simulink model "CF017A_GmVehPwrMod"  (R2013b)
settings: Solver=FixedStepDiscrete  SolverMode=SingleTasking  StartTime=0.0  StopTime=2  FixedStep=0.002  RelTol=1e-3
values from neighbouring files (symbols this model uses):
  ASSIKEEPMINIDX_CNT_U16 = DataDict.Constant    [CF017A_GmVehPwrMod_DataDict.m]
  BUSOFFHISPDIDX_CNT_U16 = DataDict.Constant    [CF017A_GmVehPwrMod_DataDict.m]
  CNTTOSEC_ULS_U32 = DataDict.Constant    [CF017A_GmVehPwrMod_DataDict.m]
  ENGRUNACTVIDX_CNT_U16 = DataDict.Constant    [CF017A_GmVehPwrMod_DataDict.m]
  GmVehPwrModHwTqMinKeepAssi = DataDict.Calibration    [CF017A_GmVehPwrMod_DataDict.m]
  GmVehPwrModHwTqMinKeepTmr = DataDict.Calibration    [CF017A_GmVehPwrMod_DataDict.m]
  GmVehPwrModOperRampRate = DataDict.Calibration    [CF017A_GmVehPwrMod_DataDict.m]
  GMVEHPWRMODSYSSTREQENA_CNT_LOGL = DataDict.Constant    [CF017A_GmVehPwrMod_DataDict.m]
  GMVEHPWRMODVAREFF_CNT_LOGL = DataDict.Constant    [CF017A_GmVehPwrMod_DataDict.m]
  GmVehPwrModVehSpdAssiOnMin = DataDict.Calibration    [CF017A_GmVehPwrMod_DataDict.m]
  GmVehPwrModVehSpdMinKeepAssi = DataDict.Calibration    [CF017A_GmVehPwrMod_DataDict.m]
  GPIOMCUENAIDX_CNT_U16 = DataDict.Constant    [CF017A_GmVehPwrMod_DataDict.m]
  KEEPASSIIDX_CNT_U16 = DataDict.Constant    [CF017A_GmVehPwrMod_DataDict.m]
  MSG0C9MISSIDX_CNT_U16 = DataDict.Constant    [CF017A_GmVehPwrMod_DataDict.m]
  MSG1F1MISSIDX_CNT_U16 = DataDict.Constant    [CF017A_GmVehPwrMod_DataDict.m]
  SYSPWRMODRUNIDX_CNT_U16 = DataDict.Constant    [CF017A_GmVehPwrMod_DataDict.m]
  VEHSPDSNSRVLDIDX_CNT_U16 = DataDict.Constant    [CF017A_GmVehPwrMod_DataDict.m]
libraries: simulink x2, NxtrLim x2, NxtrAbslt x1
(part 4 of 4)

== system CF017A_GmVehPwrMod/GmVehPwrMod/GmVehPwrModPer1/SysStReqEna_LookupTbl_KeepOn_OnToOff/KeepAssi_Bit0/Bit0_1 ==
  Action Port : ActionPort  ActionType=then
  Constant : Constant  Value=KEEPASSIIDX_CNT_U16  OutDataTypeStr=uint16
  CopyRight2 : Subsystem  Description=|  mask(Copyright Information){none=on}
      | Copyright info block.                                               
      |                                                                     
      | Place copyright information at the top of every subsystem in design.
      mask prompts: none "No parameters"
      mask help: Place copyright information at the top of every subsystem in design.
      mask Display:
      | NxtrConf = 'Nexteer Confidential';
      | 
      | sys = bdroot; %handle for the current model ("system")
      | first = get_param(sys,'Created');
      | if(isempty(first))
      |     first = datestr(now,'yyyy');
      | else
      |     first = first(end-3:end);  %year is last four digits
      | end
      | 
      | last = get_param(sys,'LastModifiedDate');
      | if isempty(last)
      |     last = datestr(now,'yyyy');
      | else
      |     last = last(end-3:end);
      | end
      | 
      | if strcmp(first,last)
      |     fprintf('%s -- Copyright %s Nexteer',NxtrConf,first)
      | else
      |     fprintf('%s -- %s%s- %s Nexteer',NxtrConf,char(169),first,last)
      | end
  Bit0Sts : Outport
  wires:
  Constant/1 -> Bit0Sts/1

== system CF017A_GmVehPwrMod/GmVehPwrMod/GmVehPwrModPer1/SysStReqEna_LookupTbl_KeepOn_OnToOff/KeepAssi_Bit0/CopyRight2 ==

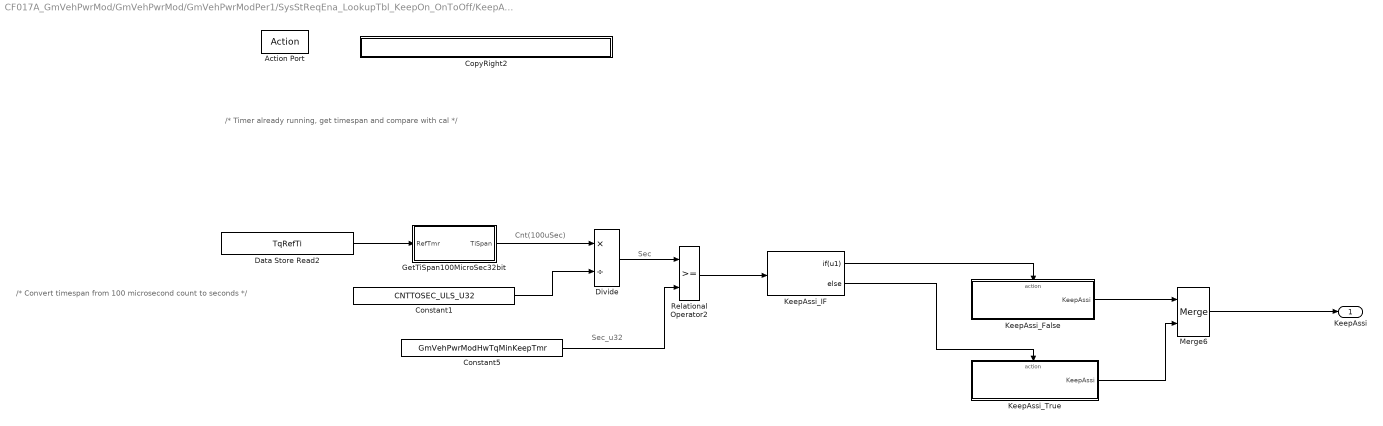
== system CF017A_GmVehPwrMod/GmVehPwrMod/GmVehPwrModPer1/SysStReqEna_LookupTbl_KeepOn_OnToOff/KeepAssi_HwTqTmr/Get_SpanTi ==
  note: Sec
  note: Cnt(100uSec)
  note: Sec_u32
  note: /* Timer already running, get timespan and compare with cal */
  note: /* Convert timespan from 100 microsecond count to seconds */
  Action Port : ActionPort  ActionType=elseif
  Constant1 : Constant  RequirementInfo={} %GIDa_aa9cc0f8_f214_4efc_ab36_0ac5a280fabf  Value=CNTTOSEC_ULS_U32  OutDataTypeStr=uint32
      settings: AttributesFormatString=%<OutDataTypeStr>
  Constant5 : Constant  RequirementInfo={} %GIDa_69eca624_6dc5_4cb0_ae9b_e1684d9a1446  Value=GmVehPwrModHwTqMinKeepTmr  OutDataTypeStr=uint32
      settings: AttributesFormatString=%<OutDataTypeStr>
  CopyRight2 : Subsystem  Description=|  mask(Copyright Information){none=on}
      | Copyright info block.                                               
      |                                                                     
      | Place copyright information at the top of every subsystem in design.
      mask prompts: none "No parameters"
      mask help: Place copyright information at the top of every subsystem in design.
      mask Display:
      | NxtrConf = 'Nexteer Confidential';
      | 
      | sys = bdroot; %handle for the current model ("system")
      | first = get_param(sys,'Created');
      | if(isempty(first))
      |     first = datestr(now,'yyyy');
      | else
      |     first = first(end-3:end);  %year is last four digits
      | end
      | 
      | last = get_param(sys,'LastModifiedDate');
      | if isempty(last)
      |     last = datestr(now,'yyyy');
      | else
      |     last = last(end-3:end);
      | end
      | 
      | if strcmp(first,last)
      |     fprintf('%s -- Copyright %s Nexteer',NxtrConf,first)
      | else
      |     fprintf('%s -- %s%s- %s Nexteer',NxtrConf,char(169),first,last)
      | end
  Data Store Read2 : DataStoreRead  DataStoreName=TqRefTi
  Divide : Product  Inputs=*/
  GetTiSpan100MicroSec32bit : Subsystem
  KeepAssi_False : Subsystem  RequirementInfo={} %GIDa_fe66f275_3ea7_40ce_bfac_a984a6fb9f78  TreatAsAtomicUnit=on
  KeepAssi_IF : If  RequirementInfo={} %GIDa_702726b2_9a9c_48b8_b9c7_15ecbfb5f8b5  IfExpression=u1
      settings: AttributesFormatString=%<Priority>
  KeepAssi_True : Subsystem  RequirementInfo={} %GIDa_583d1404_53f3_46f6_93fc_f6a44d321467  TreatAsAtomicUnit=on
  Merge6 : Merge  RequirementInfo={} %GIDa_2056328d_8088_4a66_9c76_ebdd3fb75faf
  Relational Operator2 : RelationalOperator  OutDataTypeStr=boolean
  "KeepAssi " : Outport  RequirementInfo={} %GIDa_500dc0bc_1ae5_4157_a4dd_5d2ae0a6ca5d
  wires:
  Data Store Read2/1 -> GetTiSpan100MicroSec32bit/1(RefTmr)
  Constant5/1 -> Relational Operator2/2
  GetTiSpan100MicroSec32bit/1(TiSpan) -> Divide/1
  Relational Operator2/1 -> KeepAssi_IF/1
  KeepAssi_IF/1 -> KeepAssi_False/Action
  KeepAssi_IF/2 -> KeepAssi_True/Action
  KeepAssi_False/1("KeepAssi ") -> Merge6/1
  KeepAssi_True/1("KeepAssi ") -> Merge6/2
  Constant1/1 -> Divide/2
  Divide/1 -> Relational Operator2/1
  Merge6/1 -> "KeepAssi "/1

== system CF017A_GmVehPwrMod/GmVehPwrMod/GmVehPwrModPer1/SysStReqEna_LookupTbl_KeepOn_OnToOff/KeepAssi_HwTqTmr/Stop_Tmr ==
  note: /* * Turn timer off since absolute value of handwheel torque is no longer less than HwTqMinKeepAssi cal. */
  Action Port : ActionPort  ActionType=else
  Constant1 : Constant  RequirementInfo={} %GIDa_143b7973_8004_4f87_9c2d_0949d74a0751  Value=false  OutDataTypeStr=boolean
      settings: AttributesFormatString=%<OutDataTypeStr>
  Constant4 : Constant  RequirementInfo={} %GIDa_c94d2a82_6aa0_4b23_8705_fa1f20d4de3f  Value=true  OutDataTypeStr=boolean
      settings: AttributesFormatString=%<OutDataTypeStr>
  CopyRight2 : Subsystem  Description=|  mask(Copyright Information){none=on}
      | Copyright info block.                                               
      |                                                                     
      | Place copyright information at the top of every subsystem in design.
      mask prompts: none "No parameters"
      mask help: Place copyright information at the top of every subsystem in design.
      mask Display:
      | NxtrConf = 'Nexteer Confidential';
      | 
      | sys = bdroot; %handle for the current model ("system")
      | first = get_param(sys,'Created');
      | if(isempty(first))
      |     first = datestr(now,'yyyy');
      | else
      |     first = first(end-3:end);  %year is last four digits
      | end
      | 
      | last = get_param(sys,'LastModifiedDate');
      | if isempty(last)
      |     last = datestr(now,'yyyy');
      | else
      |     last = last(end-3:end);
      | end
      | 
      | if strcmp(first,last)
      |     fprintf('%s -- Copyright %s Nexteer',NxtrConf,first)
      | else
      |     fprintf('%s -- %s%s- %s Nexteer',NxtrConf,char(169),first,last)
      | end
  Data Store Write2 : DataStoreWrite  DataStoreName=TqRefTiActv
      settings: AttributesFormatString=%<Priority>
  "KeepAssi " : Outport  RequirementInfo={} %GIDa_99310702_14e0_41e3_9d7b_f2280936931a
  wires:
  Constant1/1 -> Data Store Write2/1
  Constant4/1 -> "KeepAssi "/1

== system CF017A_GmVehPwrMod/GmVehPwrMod/GmVehPwrModPer1/SysStReqEna_LookupTbl_KeepOn_OnToOff/KeepAssi_HwTqTmr/Tmr_Strt ==
  note: /* HwTq dipped below minimum needed to keep assist and timer not yet active so start the timer now. */
  Action Port : ActionPort  ActionType=then
  Constant1 : Constant  RequirementInfo={} %GIDa_b7fdb1af_31c1_494c_99c2_7093c5cc2f63  Value=true  OutDataTypeStr=boolean
      settings: AttributesFormatString=%<OutDataTypeStr>
  Constant4 : Constant  RequirementInfo={} %GIDa_ab99e30b_c1a7_4330_836d_a1e94e7d5cba  Value=true  OutDataTypeStr=boolean
      settings: AttributesFormatString=%<OutDataTypeStr>
  CopyRight2 : Subsystem  Description=|  mask(Copyright Information){none=on}
      | Copyright info block.                                               
      |                                                                     
      | Place copyright information at the top of every subsystem in design.
      mask prompts: none "No parameters"
      mask help: Place copyright information at the top of every subsystem in design.
      mask Display:
      | NxtrConf = 'Nexteer Confidential';
      | 
      | sys = bdroot; %handle for the current model ("system")
      | first = get_param(sys,'Created');
      | if(isempty(first))
      |     first = datestr(now,'yyyy');
      | else
      |     first = first(end-3:end);  %year is last four digits
      | end
      | 
      | last = get_param(sys,'LastModifiedDate');
      | if isempty(last)
      |     last = datestr(now,'yyyy');
      | else
      |     last = last(end-3:end);
      | end
      | 
      | if strcmp(first,last)
      |     fprintf('%s -- Copyright %s Nexteer',NxtrConf,first)
      | else
      |     fprintf('%s -- %s%s- %s Nexteer',NxtrConf,char(169),first,last)
      | end
  Data Store Write1 : DataStoreWrite  DataStoreName=TqRefTi
      settings: AttributesFormatString=%<Priority>
  Data Store Write2 : DataStoreWrite  DataStoreName=TqRefTiActv
      settings: AttributesFormatString=%<Priority>
  GetRefTmr100MicroSec32bit1 : Subsystem
  "KeepAssi " : Outport  RequirementInfo={} %GIDa_aae598dd_8360_4797_8d07_5dbb83386652
  wires:
  Constant4/1 -> Data Store Write2/1
  GetRefTmr100MicroSec32bit1/1(RefTmr) -> Data Store Write1/1
  Constant1/1 -> "KeepAssi "/1

== system CF017A_GmVehPwrMod/GmVehPwrMod/GmVehPwrModPer1/SysStReqEna_LookupTbl_KeepOn_OnToOff/Msg0C9Missa_Bit4/Bit4_0 ==
  Action Port : ActionPort  ActionType=else
  Constant1 : Constant  Value=0  OutDataTypeStr=uint16
      settings: AttributesFormatString=%<OutDataTypeStr>
  CopyRight2 : Subsystem  Description=|  mask(Copyright Information){none=on}
      | Copyright info block.                                               
      |                                                                     
      | Place copyright information at the top of every subsystem in design.
      mask prompts: none "No parameters"
      mask help: Place copyright information at the top of every subsystem in design.
      mask Display:
      | NxtrConf = 'Nexteer Confidential';
      | 
      | sys = bdroot; %handle for the current model ("system")
      | first = get_param(sys,'Created');
      | if(isempty(first))
      |     first = datestr(now,'yyyy');
      | else
      |     first = first(end-3:end);  %year is last four digits
      | end
      | 
      | last = get_param(sys,'LastModifiedDate');
      | if isempty(last)
      |     last = datestr(now,'yyyy');
      | else
      |     last = last(end-3:end);
      | end
      | 
      | if strcmp(first,last)
      |     fprintf('%s -- Copyright %s Nexteer',NxtrConf,first)
      | else
      |     fprintf('%s -- %s%s- %s Nexteer',NxtrConf,char(169),first,last)
      | end
  Bit4Sts : Outport
  wires:
  Constant1/1 -> Bit4Sts/1

== system CF017A_GmVehPwrMod/GmVehPwrMod/GmVehPwrModPer1/SysStReqEna_LookupTbl_KeepOn_OnToOff/Msg0C9Missa_Bit4/Bit4_16 ==
  Action Port : ActionPort  ActionType=then
  Constant : Constant  Value=MSG0C9MISSIDX_CNT_U16  OutDataTypeStr=uint16
  CopyRight2 : Subsystem  Description=|  mask(Copyright Information){none=on}
      | Copyright info block.                                               
      |                                                                     
      | Place copyright information at the top of every subsystem in design.
      mask prompts: none "No parameters"
      mask help: Place copyright information at the top of every subsystem in design.
      mask Display:
      | NxtrConf = 'Nexteer Confidential';
      | 
      | sys = bdroot; %handle for the current model ("system")
      | first = get_param(sys,'Created');
      | if(isempty(first))
      |     first = datestr(now,'yyyy');
      | else
      |     first = first(end-3:end);  %year is last four digits
      | end
      | 
      | last = get_param(sys,'LastModifiedDate');
      | if isempty(last)
      |     last = datestr(now,'yyyy');
      | else
      |     last = last(end-3:end);
      | end
      | 
      | if strcmp(first,last)
      |     fprintf('%s -- Copyright %s Nexteer',NxtrConf,first)
      | else
      |     fprintf('%s -- %s%s- %s Nexteer',NxtrConf,char(169),first,last)
      | end
  Bit4Sts : Outport
  wires:
  Constant/1 -> Bit4Sts/1

== system CF017A_GmVehPwrMod/GmVehPwrMod/GmVehPwrModPer1/SysStReqEna_LookupTbl_KeepOn_OnToOff/Msg0C9Missa_Bit4/CopyRight2 ==

== system CF017A_GmVehPwrMod/GmVehPwrMod/GmVehPwrModPer1/SysStReqEna_LookupTbl_KeepOn_OnToOff/Msg1F1Miss_Bit2/Bit2_0 ==
  Action Port : ActionPort  ActionType=else
  Constant1 : Constant  Value=0  OutDataTypeStr=uint16
      settings: AttributesFormatString=%<OutDataTypeStr>
  CopyRight2 : Subsystem  Description=|  mask(Copyright Information){none=on}
      | Copyright info block.                                               
      |                                                                     
      | Place copyright information at the top of every subsystem in design.
      mask prompts: none "No parameters"
      mask help: Place copyright information at the top of every subsystem in design.
      mask Display:
      | NxtrConf = 'Nexteer Confidential';
      | 
      | sys = bdroot; %handle for the current model ("system")
      | first = get_param(sys,'Created');
      | if(isempty(first))
      |     first = datestr(now,'yyyy');
      | else
      |     first = first(end-3:end);  %year is last four digits
      | end
      | 
      | last = get_param(sys,'LastModifiedDate');
      | if isempty(last)
      |     last = datestr(now,'yyyy');
      | else
      |     last = last(end-3:end);
      | end
      | 
      | if strcmp(first,last)
      |     fprintf('%s -- Copyright %s Nexteer',NxtrConf,first)
      | else
      |     fprintf('%s -- %s%s- %s Nexteer',NxtrConf,char(169),first,last)
      | end
  Bit2Sts : Outport
  wires:
  Constant1/1 -> Bit2Sts/1

== system CF017A_GmVehPwrMod/GmVehPwrMod/GmVehPwrModPer1/SysStReqEna_LookupTbl_KeepOn_OnToOff/Msg1F1Miss_Bit2/Bit2_4 ==
  Action Port : ActionPort  ActionType=then
  Constant : Constant  Value=MSG1F1MISSIDX_CNT_U16  OutDataTypeStr=uint16
  CopyRight2 : Subsystem  Description=|  mask(Copyright Information){none=on}
      | Copyright info block.                                               
      |                                                                     
      | Place copyright information at the top of every subsystem in design.
      mask prompts: none "No parameters"
      mask help: Place copyright information at the top of every subsystem in design.
      mask Display:
      | NxtrConf = 'Nexteer Confidential';
      | 
      | sys = bdroot; %handle for the current model ("system")
      | first = get_param(sys,'Created');
      | if(isempty(first))
      |     first = datestr(now,'yyyy');
      | else
      |     first = first(end-3:end);  %year is last four digits
      | end
      | 
      | last = get_param(sys,'LastModifiedDate');
      | if isempty(last)
      |     last = datestr(now,'yyyy');
      | else
      |     last = last(end-3:end);
      | end
      | 
      | if strcmp(first,last)
      |     fprintf('%s -- Copyright %s Nexteer',NxtrConf,first)
      | else
      |     fprintf('%s -- %s%s- %s Nexteer',NxtrConf,char(169),first,last)
      | end
  Bit2Sts : Outport
  wires:
  Constant/1 -> Bit2Sts/1

== system CF017A_GmVehPwrMod/GmVehPwrMod/GmVehPwrModPer1/SysStReqEna_LookupTbl_KeepOn_OnToOff/Msg1F1Miss_Bit2/CopyRight2 ==

== system CF017A_GmVehPwrMod/GmVehPwrMod/GmVehPwrModPer1/SysStReqEna_LookupTbl_KeepOn_OnToOff/SysPwrModRun_Bit7/Bit7_0 ==
  Action Port : ActionPort  ActionType=else
  Constant1 : Constant  Value=0  OutDataTypeStr=uint16
      settings: AttributesFormatString=%<OutDataTypeStr>
  CopyRight2 : Subsystem  Description=|  mask(Copyright Information){none=on}
      | Copyright info block.                                               
      |                                                                     
      | Place copyright information at the top of every subsystem in design.
      mask prompts: none "No parameters"
      mask help: Place copyright information at the top of every subsystem in design.
      mask Display:
      | NxtrConf = 'Nexteer Confidential';
      | 
      | sys = bdroot; %handle for the current model ("system")
      | first = get_param(sys,'Created');
      | if(isempty(first))
      |     first = datestr(now,'yyyy');
      | else
      |     first = first(end-3:end);  %year is last four digits
      | end
      | 
      | last = get_param(sys,'LastModifiedDate');
      | if isempty(last)
      |     last = datestr(now,'yyyy');
      | else
      |     last = last(end-3:end);
      | end
      | 
      | if strcmp(first,last)
      |     fprintf('%s -- Copyright %s Nexteer',NxtrConf,first)
      | else
      |     fprintf('%s -- %s%s- %s Nexteer',NxtrConf,char(169),first,last)
      | end
  Bit7Sts : Outport
  wires:
  Constant1/1 -> Bit7Sts/1

== system CF017A_GmVehPwrMod/GmVehPwrMod/GmVehPwrModPer1/SysStReqEna_LookupTbl_KeepOn_OnToOff/SysPwrModRun_Bit7/Bit7_128 ==
  Action Port : ActionPort  ActionType=then
  Constant : Constant  Value=SYSPWRMODRUNIDX_CNT_U16  OutDataTypeStr=uint16
  CopyRight2 : Subsystem  Description=|  mask(Copyright Information){none=on}
      | Copyright info block.                                               
      |                                                                     
      | Place copyright information at the top of every subsystem in design.
      mask prompts: none "No parameters"
      mask help: Place copyright information at the top of every subsystem in design.
      mask Display:
      | NxtrConf = 'Nexteer Confidential';
      | 
      | sys = bdroot; %handle for the current model ("system")
      | first = get_param(sys,'Created');
      | if(isempty(first))
      |     first = datestr(now,'yyyy');
      | else
      |     first = first(end-3:end);  %year is last four digits
      | end
      | 
      | last = get_param(sys,'LastModifiedDate');
      | if isempty(last)
      |     last = datestr(now,'yyyy');
      | else
      |     last = last(end-3:end);
      | end
      | 
      | if strcmp(first,last)
      |     fprintf('%s -- Copyright %s Nexteer',NxtrConf,first)
      | else
      |     fprintf('%s -- %s%s- %s Nexteer',NxtrConf,char(169),first,last)
      | end
  Bit7Sts : Outport
  wires:
  Constant/1 -> Bit7Sts/1

== system CF017A_GmVehPwrMod/GmVehPwrMod/GmVehPwrModPer1/SysStReqEna_LookupTbl_KeepOn_OnToOff/SysPwrModRun_Bit7/CopyRight2 ==

== system CF017A_GmVehPwrMod/GmVehPwrMod/GmVehPwrModPer1/SysStReqEna_LookupTbl_KeepOn_OnToOff/VehSpdSnsrVld_Bit3/Bit3_0 ==
  Action Port : ActionPort  ActionType=else
  Constant1 : Constant  Value=0  OutDataTypeStr=uint16
      settings: AttributesFormatString=%<OutDataTypeStr>
  CopyRight2 : Subsystem  Description=|  mask(Copyright Information){none=on}
      | Copyright info block.                                               
      |                                                                     
      | Place copyright information at the top of every subsystem in design.
      mask prompts: none "No parameters"
      mask help: Place copyright information at the top of every subsystem in design.
      mask Display:
      | NxtrConf = 'Nexteer Confidential';
      | 
      | sys = bdroot; %handle for the current model ("system")
      | first = get_param(sys,'Created');
      | if(isempty(first))
      |     first = datestr(now,'yyyy');
      | else
      |     first = first(end-3:end);  %year is last four digits
      | end
      | 
      | last = get_param(sys,'LastModifiedDate');
      | if isempty(last)
      |     last = datestr(now,'yyyy');
      | else
      |     last = last(end-3:end);
      | end
      | 
      | if strcmp(first,last)
      |     fprintf('%s -- Copyright %s Nexteer',NxtrConf,first)
      | else
      |     fprintf('%s -- %s%s- %s Nexteer',NxtrConf,char(169),first,last)
      | end
  Bit3Sts : Outport
  wires:
  Constant1/1 -> Bit3Sts/1

== system CF017A_GmVehPwrMod/GmVehPwrMod/GmVehPwrModPer1/SysStReqEna_LookupTbl_KeepOn_OnToOff/VehSpdSnsrVld_Bit3/Bit3_8 ==
  Action Port : ActionPort  ActionType=then
  Constant : Constant  Value=VEHSPDSNSRVLDIDX_CNT_U16  OutDataTypeStr=uint16
  CopyRight2 : Subsystem  Description=|  mask(Copyright Information){none=on}
      | Copyright info block.                                               
      |                                                                     
      | Place copyright information at the top of every subsystem in design.
      mask prompts: none "No parameters"
      mask help: Place copyright information at the top of every subsystem in design.
      mask Display:
      | NxtrConf = 'Nexteer Confidential';
      | 
      | sys = bdroot; %handle for the current model ("system")
      | first = get_param(sys,'Created');
      | if(isempty(first))
      |     first = datestr(now,'yyyy');
      | else
      |     first = first(end-3:end);  %year is last four digits
      | end
      | 
      | last = get_param(sys,'LastModifiedDate');
      | if isempty(last)
      |     last = datestr(now,'yyyy');
      | else
      |     last = last(end-3:end);
      | end
      | 
      | if strcmp(first,last)
      |     fprintf('%s -- Copyright %s Nexteer',NxtrConf,first)
      | else
      |     fprintf('%s -- %s%s- %s Nexteer',NxtrConf,char(169),first,last)
      | end
  Bit3Sts : Outport
  wires:
  Constant/1 -> Bit3Sts/1

== system CF017A_GmVehPwrMod/GmVehPwrMod/GmVehPwrModPer1/SysStReqEna_LookupTbl_KeepOn_OnToOff/VehSpdSnsrVld_Bit3/CopyRight2 ==

== system CF017A_GmVehPwrMod/GmVehPwrMod/GmVehPwrModPer1/TqCmdSca_VehSpdEna_Sub/Set_SpdEna_False/CopyRight2 ==

== system CF017A_GmVehPwrMod/GmVehPwrMod/GmVehPwrModPer1/TqCmdSca_VehSpdEna_Sub/Set_SpdEna_True/CopyRight2 ==

== system CF017A_GmVehPwrMod/GmVehPwrMod/GmVehPwrModPer1/TqCmdSca_VehSpdEna_Sub/TqCmdSca_0/CopyRight2 ==

== system CF017A_GmVehPwrMod/GmVehPwrMod/GmVehPwrModPer1/TqCmdSca_VehSpdEna_Sub/TqCmdSca_1/CopyRight2 ==

== system CF017A_GmVehPwrMod/GmVehPwrMod/GmVehPwrModPer1/SysStReqEna_LookupTbl_KeepOn_OnToOff/AssiKeepMin_Bit5/Bit5_0/CopyRight2 ==

== system CF017A_GmVehPwrMod/GmVehPwrMod/GmVehPwrModPer1/SysStReqEna_LookupTbl_KeepOn_OnToOff/AssiKeepMin_Bit5/Bit5_32/CopyRight2 ==

== system CF017A_GmVehPwrMod/GmVehPwrMod/GmVehPwrModPer1/SysStReqEna_LookupTbl_KeepOn_OnToOff/BusOffHiSpd_Bit1/Bit1_0/CopyRight2 ==

== system CF017A_GmVehPwrMod/GmVehPwrMod/GmVehPwrModPer1/SysStReqEna_LookupTbl_KeepOn_OnToOff/BusOffHiSpd_Bit1/Bit1_2/CopyRight2 ==

== system CF017A_GmVehPwrMod/GmVehPwrMod/GmVehPwrModPer1/SysStReqEna_LookupTbl_KeepOn_OnToOff/EngRunActv_Bit6/Bit6_0/CopyRight2 ==

== system CF017A_GmVehPwrMod/GmVehPwrMod/GmVehPwrModPer1/SysStReqEna_LookupTbl_KeepOn_OnToOff/EngRunActv_Bit6/Bit6_64/CopyRight2 ==

== system CF017A_GmVehPwrMod/GmVehPwrMod/GmVehPwrModPer1/SysStReqEna_LookupTbl_KeepOn_OnToOff/GpioMcuEna_Bit8/Bit8_0/CopyRight2 ==

== system CF017A_GmVehPwrMod/GmVehPwrMod/GmVehPwrModPer1/SysStReqEna_LookupTbl_KeepOn_OnToOff/GpioMcuEna_Bit8/Bit8_256/CopyRight2 ==

== system CF017A_GmVehPwrMod/GmVehPwrMod/GmVehPwrModPer1/SysStReqEna_LookupTbl_KeepOn_OnToOff/KeepAssi_Bit0/Bit0_0/CopyRight2 ==

== system CF017A_GmVehPwrMod/GmVehPwrMod/GmVehPwrModPer1/SysStReqEna_LookupTbl_KeepOn_OnToOff/KeepAssi_Bit0/Bit0_1/CopyRight2 ==

== system CF017A_GmVehPwrMod/GmVehPwrMod/GmVehPwrModPer1/SysStReqEna_LookupTbl_KeepOn_OnToOff/KeepAssi_HwTqTmr/Get_SpanTi/CopyRight2 ==

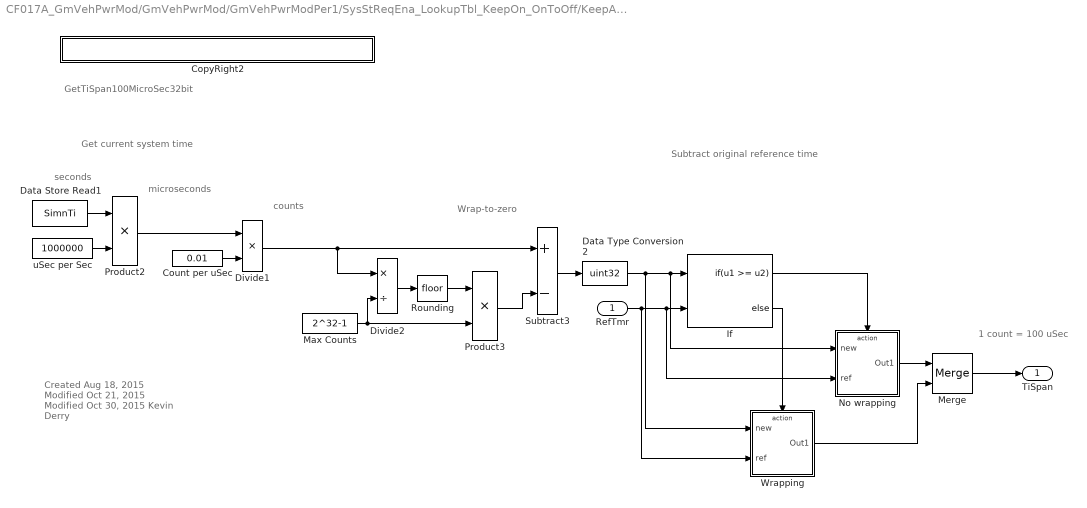
== system CF017A_GmVehPwrMod/GmVehPwrMod/GmVehPwrModPer1/SysStReqEna_LookupTbl_KeepOn_OnToOff/KeepAssi_HwTqTmr/Get_SpanTi/GetTiSpan100MicroSec32bit ==
  note: Created Aug 18, 2015
      | Modified Oct 21, 2015
      | Modified Oct 30, 2015
      | Kevin Derry
  note: GetTiSpan100MicroSec32bit
  note: Get current system time
  note: 1 count = 100 uSec
  note: Wrap-to-zero
  note: counts
  note: microseconds
  note: seconds
  note: Subtract original reference time
  RefTmr : Inport
  CopyRight2 : Subsystem  Description=|  mask(Copyright Information){none=on}
      | Copyright info block.                                               
      |                                                                     
      | Place copyright information at the top of every subsystem in design.
      mask prompts: none "No parameters"
      mask help: Place copyright information at the top of every subsystem in design.
      mask Display:
      | NxtrConf = 'Nexteer Confidential';
      | 
      | sys = bdroot; %handle for the current model ("system")
      | first = get_param(sys,'Created');
      | if(isempty(first))
      |     first = datestr(now,'yyyy');
      | else
      |     first = first(end-3:end);  %year is last four digits
      | end
      | 
      | last = get_param(sys,'LastModifiedDate');
      | if isempty(last)
      |     last = datestr(now,'yyyy');
      | else
      |     last = last(end-3:end);
      | end
      | 
      | if strcmp(first,last)
      |     fprintf('%s -- Copyright %s Nexteer',NxtrConf,first)
      | else
      |     fprintf('%s -- %s%s- %s Nexteer',NxtrConf,char(169),first,last)
      | end
  Count per uSec : Constant  Value=0.01
  Data Store Read1 : DataStoreRead  DataStoreName=SimnTi
  Data Type Conversion2 : DataTypeConversion  OutDataTypeStr=uint32
  Divide1 : Product  Inputs=**
  Divide2 : Product  Inputs=*/
  If : If  NumInputs=2  IfExpression=u1 >= u2
  Max Counts : Constant  Value=2^32-1
  Merge : Merge
  No wrapping : Subsystem  TreatAsAtomicUnit=on
  Product2 : Product
  Product3 : Product
  Rounding : Rounding
  Subtract3 : Sum  Inputs=+-
  Wrapping : Subsystem  TreatAsAtomicUnit=on
  uSec per Sec : Constant  Value=1000000
  TiSpan : Outport
  wires:
  Data Type Conversion2/1 -> Wrapping/1(new), No wrapping/1(new), If/1
  RefTmr/1 -> Wrapping/2(ref), No wrapping/2(ref), If/2
  Merge/1 -> TiSpan/1
  uSec per Sec/1 -> Product2/2
  Count per uSec/1 -> Divide1/2
  Data Store Read1/1 -> Product2/1
  Product2/1 -> Divide1/1
  Divide1/1 -> Subtract3/1, Divide2/1
  Max Counts/1 -> Product3/2, Divide2/2
  Divide2/1 -> Rounding/1
  Rounding/1 -> Product3/1
  Subtract3/1 -> Data Type Conversion2/1
  Product3/1 -> Subtract3/2
  If/1 -> No wrapping/Action
  If/2 -> Wrapping/Action
  No wrapping/1(Out1) -> Merge/1
  Wrapping/1(Out1) -> Merge/2

== system CF017A_GmVehPwrMod/GmVehPwrMod/GmVehPwrModPer1/SysStReqEna_LookupTbl_KeepOn_OnToOff/KeepAssi_HwTqTmr/Get_SpanTi/KeepAssi_False ==
  Action Port : ActionPort  ActionType=then
  Constant4 : Constant  RequirementInfo={} %GIDa_fcf96f1f_2576_4238_bfd9_3130f9c8bd09  Value=false  OutDataTypeStr=boolean
      settings: AttributesFormatString=%<OutDataTypeStr>
  CopyRight2 : Subsystem  Description=|  mask(Copyright Information){none=on}
      | Copyright info block.                                               
      |                                                                     
      | Place copyright information at the top of every subsystem in design.
      mask prompts: none "No parameters"
      mask help: Place copyright information at the top of every subsystem in design.
      mask Display:
      | NxtrConf = 'Nexteer Confidential';
      | 
      | sys = bdroot; %handle for the current model ("system")
      | first = get_param(sys,'Created');
      | if(isempty(first))
      |     first = datestr(now,'yyyy');
      | else
      |     first = first(end-3:end);  %year is last four digits
      | end
      | 
      | last = get_param(sys,'LastModifiedDate');
      | if isempty(last)
      |     last = datestr(now,'yyyy');
      | else
      |     last = last(end-3:end);
      | end
      | 
      | if strcmp(first,last)
      |     fprintf('%s -- Copyright %s Nexteer',NxtrConf,first)
      | else
      |     fprintf('%s -- %s%s- %s Nexteer',NxtrConf,char(169),first,last)
      | end
  "KeepAssi " : Outport  RequirementInfo={} %GIDa_d54755f6_8567_45f1_a4bd_9b092306dc34
  wires:
  Constant4/1 -> "KeepAssi "/1

== system CF017A_GmVehPwrMod/GmVehPwrMod/GmVehPwrModPer1/SysStReqEna_LookupTbl_KeepOn_OnToOff/KeepAssi_HwTqTmr/Get_SpanTi/KeepAssi_True ==
  Action Port : ActionPort  ActionType=else
  Constant4 : Constant  RequirementInfo={} %GIDa_db190035_c479_470f_a7b3_5a0a50ad4caf  Value=true  OutDataTypeStr=boolean
      settings: AttributesFormatString=%<OutDataTypeStr>
  CopyRight2 : Subsystem  Description=|  mask(Copyright Information){none=on}
      | Copyright info block.                                               
      |                                                                     
      | Place copyright information at the top of every subsystem in design.
      mask prompts: none "No parameters"
      mask help: Place copyright information at the top of every subsystem in design.
      mask Display:
      | NxtrConf = 'Nexteer Confidential';
      | 
      | sys = bdroot; %handle for the current model ("system")
      | first = get_param(sys,'Created');
      | if(isempty(first))
      |     first = datestr(now,'yyyy');
      | else
      |     first = first(end-3:end);  %year is last four digits
      | end
      | 
      | last = get_param(sys,'LastModifiedDate');
      | if isempty(last)
      |     last = datestr(now,'yyyy');
      | else
      |     last = last(end-3:end);
      | end
      | 
      | if strcmp(first,last)
      |     fprintf('%s -- Copyright %s Nexteer',NxtrConf,first)
      | else
      |     fprintf('%s -- %s%s- %s Nexteer',NxtrConf,char(169),first,last)
      | end
  "KeepAssi " : Outport  RequirementInfo={} %GIDa_2b66be95_6046_4d59_8c00_9ed1aa99c759
  wires:
  Constant4/1 -> "KeepAssi "/1

== system CF017A_GmVehPwrMod/GmVehPwrMod/GmVehPwrModPer1/SysStReqEna_LookupTbl_KeepOn_OnToOff/KeepAssi_HwTqTmr/Stop_Tmr/CopyRight2 ==

== system CF017A_GmVehPwrMod/GmVehPwrMod/GmVehPwrModPer1/SysStReqEna_LookupTbl_KeepOn_OnToOff/KeepAssi_HwTqTmr/Tmr_Strt/CopyRight2 ==

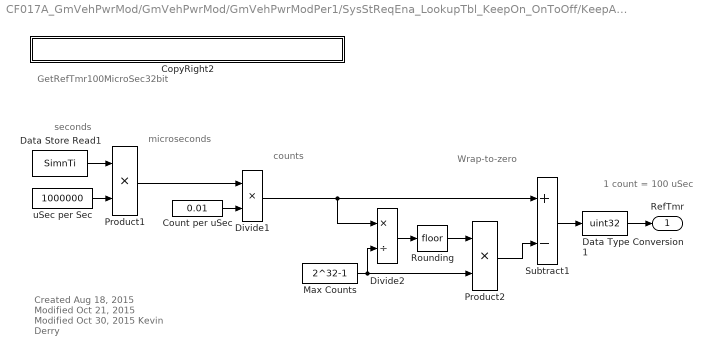
== system CF017A_GmVehPwrMod/GmVehPwrMod/GmVehPwrModPer1/SysStReqEna_LookupTbl_KeepOn_OnToOff/KeepAssi_HwTqTmr/Tmr_Strt/GetRefTmr100MicroSec32bit1 ==
  note: Created Aug 18, 2015
      | Modified Oct 21, 2015
      | Modified Oct 30, 2015
      | Kevin Derry
  note: GetRefTmr100MicroSec32bit
  note: Wrap-to-zero
  note: counts
  note: microseconds
  note: seconds
  note: 1 count = 100 uSec
  CopyRight2 : Subsystem  Description=|  mask(Copyright Information){none=on}
      | Copyright info block.                                               
      |                                                                     
      | Place copyright information at the top of every subsystem in design.
      mask prompts: none "No parameters"
      mask help: Place copyright information at the top of every subsystem in design.
      mask Display:
      | NxtrConf = 'Nexteer Confidential';
      | 
      | sys = bdroot; %handle for the current model ("system")
      | first = get_param(sys,'Created');
      | if(isempty(first))
      |     first = datestr(now,'yyyy');
      | else
      |     first = first(end-3:end);  %year is last four digits
      | end
      | 
      | last = get_param(sys,'LastModifiedDate');
      | if isempty(last)
      |     last = datestr(now,'yyyy');
      | else
      |     last = last(end-3:end);
      | end
      | 
      | if strcmp(first,last)
      |     fprintf('%s -- Copyright %s Nexteer',NxtrConf,first)
      | else
      |     fprintf('%s -- %s%s- %s Nexteer',NxtrConf,char(169),first,last)
      | end
  Count per uSec : Constant  Value=0.01
  Data Store Read1 : DataStoreRead  DataStoreName=SimnTi
  Data Type Conversion1 : DataTypeConversion  OutDataTypeStr=uint32
  Divide1 : Product  Inputs=**
  Divide2 : Product  Inputs=*/
  Max Counts : Constant  Value=2^32-1
  Product1 : Product
  Product2 : Product
  Rounding : Rounding
  Subtract1 : Sum  Inputs=+-
  uSec per Sec : Constant  Value=1000000
  RefTmr : Outport
  wires:
  Data Store Read1/1 -> Product1/1
  Data Type Conversion1/1 -> RefTmr/1
  uSec per Sec/1 -> Product1/2
  Count per uSec/1 -> Divide1/2
  Product1/1 -> Divide1/1
  Divide1/1 -> Subtract1/1, Divide2/1
  Max Counts/1 -> Product2/2, Divide2/2
  Divide2/1 -> Rounding/1
  Rounding/1 -> Product2/1
  Subtract1/1 -> Data Type Conversion1/1
  Product2/1 -> Subtract1/2

== system CF017A_GmVehPwrMod/GmVehPwrMod/GmVehPwrModPer1/SysStReqEna_LookupTbl_KeepOn_OnToOff/Msg0C9Missa_Bit4/Bit4_0/CopyRight2 ==

== system CF017A_GmVehPwrMod/GmVehPwrMod/GmVehPwrModPer1/SysStReqEna_LookupTbl_KeepOn_OnToOff/Msg0C9Missa_Bit4/Bit4_16/CopyRight2 ==

== system CF017A_GmVehPwrMod/GmVehPwrMod/GmVehPwrModPer1/SysStReqEna_LookupTbl_KeepOn_OnToOff/Msg1F1Miss_Bit2/Bit2_0/CopyRight2 ==

== system CF017A_GmVehPwrMod/GmVehPwrMod/GmVehPwrModPer1/SysStReqEna_LookupTbl_KeepOn_OnToOff/Msg1F1Miss_Bit2/Bit2_4/CopyRight2 ==

== system CF017A_GmVehPwrMod/GmVehPwrMod/GmVehPwrModPer1/SysStReqEna_LookupTbl_KeepOn_OnToOff/SysPwrModRun_Bit7/Bit7_0/CopyRight2 ==

== system CF017A_GmVehPwrMod/GmVehPwrMod/GmVehPwrModPer1/SysStReqEna_LookupTbl_KeepOn_OnToOff/SysPwrModRun_Bit7/Bit7_128/CopyRight2 ==

== system CF017A_GmVehPwrMod/GmVehPwrMod/GmVehPwrModPer1/SysStReqEna_LookupTbl_KeepOn_OnToOff/VehSpdSnsrVld_Bit3/Bit3_0/CopyRight2 ==

== system CF017A_GmVehPwrMod/GmVehPwrMod/GmVehPwrModPer1/SysStReqEna_LookupTbl_KeepOn_OnToOff/VehSpdSnsrVld_Bit3/Bit3_8/CopyRight2 ==

== system CF017A_GmVehPwrMod/GmVehPwrMod/GmVehPwrModPer1/SysStReqEna_LookupTbl_KeepOn_OnToOff/KeepAssi_HwTqTmr/Get_SpanTi/GetTiSpan100MicroSec32bit/CopyRight2 ==

== system CF017A_GmVehPwrMod/GmVehPwrMod/GmVehPwrModPer1/SysStReqEna_LookupTbl_KeepOn_OnToOff/KeepAssi_HwTqTmr/Get_SpanTi/GetTiSpan100MicroSec32bit/No wrapping ==
  new : Inport
  ref : Inport  Port=2
  Action Port : ActionPort  ActionType=then
  CopyRight2 : Subsystem  Description=|  mask(Copyright Information){none=on}
      | Copyright info block.                                               
      |                                                                     
      | Place copyright information at the top of every subsystem in design.
      mask prompts: none "No parameters"
      mask help: Place copyright information at the top of every subsystem in design.
      mask Display:
      | NxtrConf = 'Nexteer Confidential';
      | 
      | sys = bdroot; %handle for the current model ("system")
      | first = get_param(sys,'Created');
      | if(isempty(first))
      |     first = datestr(now,'yyyy');
      | else
      |     first = first(end-3:end);  %year is last four digits
      | end
      | 
      | last = get_param(sys,'LastModifiedDate');
      | if isempty(last)
      |     last = datestr(now,'yyyy');
      | else
      |     last = last(end-3:end);
      | end
      | 
      | if strcmp(first,last)
      |     fprintf('%s -- Copyright %s Nexteer',NxtrConf,first)
      | else
      |     fprintf('%s -- %s%s- %s Nexteer',NxtrConf,char(169),first,last)
      | end
  Subtract1 : Sum  Inputs=+-
  Out1 : Outport
  wires:
  Subtract1/1 -> Out1/1
  new/1 -> Subtract1/1
  ref/1 -> Subtract1/2

== system CF017A_GmVehPwrMod/GmVehPwrMod/GmVehPwrModPer1/SysStReqEna_LookupTbl_KeepOn_OnToOff/KeepAssi_HwTqTmr/Get_SpanTi/GetTiSpan100MicroSec32bit/Wrapping ==
  new : Inport
  ref : Inport  Port=2
  Action Port : ActionPort  ActionType=else
  CopyRight2 : Subsystem  Description=|  mask(Copyright Information){none=on}
      | Copyright info block.                                               
      |                                                                     
      | Place copyright information at the top of every subsystem in design.
      mask prompts: none "No parameters"
      mask help: Place copyright information at the top of every subsystem in design.
      mask Display:
      | NxtrConf = 'Nexteer Confidential';
      | 
      | sys = bdroot; %handle for the current model ("system")
      | first = get_param(sys,'Created');
      | if(isempty(first))
      |     first = datestr(now,'yyyy');
      | else
      |     first = first(end-3:end);  %year is last four digits
      | end
      | 
      | last = get_param(sys,'LastModifiedDate');
      | if isempty(last)
      |     last = datestr(now,'yyyy');
      | else
      |     last = last(end-3:end);
      | end
      | 
      | if strcmp(first,last)
      |     fprintf('%s -- Copyright %s Nexteer',NxtrConf,first)
      | else
      |     fprintf('%s -- %s%s- %s Nexteer',NxtrConf,char(169),first,last)
      | end
  Max Counts : Constant  Value=2^32-1  OutDataTypeStr=uint32
  Subtract1 : Sum  Inputs=+-+
  Out1 : Outport
  wires:
  Subtract1/1 -> Out1/1
  Max Counts/1 -> Subtract1/1
  ref/1 -> Subtract1/2
  new/1 -> Subtract1/3

== system CF017A_GmVehPwrMod/GmVehPwrMod/GmVehPwrModPer1/SysStReqEna_LookupTbl_KeepOn_OnToOff/KeepAssi_HwTqTmr/Get_SpanTi/KeepAssi_False/CopyRight2 ==

== system CF017A_GmVehPwrMod/GmVehPwrMod/GmVehPwrModPer1/SysStReqEna_LookupTbl_KeepOn_OnToOff/KeepAssi_HwTqTmr/Get_SpanTi/KeepAssi_True/CopyRight2 ==

== system CF017A_GmVehPwrMod/GmVehPwrMod/GmVehPwrModPer1/SysStReqEna_LookupTbl_KeepOn_OnToOff/KeepAssi_HwTqTmr/Tmr_Strt/GetRefTmr100MicroSec32bit1/CopyRight2 ==

== system CF017A_GmVehPwrMod/GmVehPwrMod/GmVehPwrModPer1/SysStReqEna_LookupTbl_KeepOn_OnToOff/KeepAssi_HwTqTmr/Get_SpanTi/GetTiSpan100MicroSec32bit/No wrapping/CopyRight2 ==

== system CF017A_GmVehPwrMod/GmVehPwrMod/GmVehPwrModPer1/SysStReqEna_LookupTbl_KeepOn_OnToOff/KeepAssi_HwTqTmr/Get_SpanTi/GetTiSpan100MicroSec32bit/Wrapping/CopyRight2 ==
